simulink model "Working_Dynamics_Sparkle"  (R2018b)
settings: Solver=FixedStepAuto  StartTime=0.0  StopTime=inf  FixedStep=0.0005  RelTol=1e-3
model workspace (MAT data in the model file):
  A_mu = 10
  B_reff = 8.386
  Cz = 7766.25
  DCT_Param.Transmission.Ratios = [3.78 2.18 1.43 1.03 0.935 0.84]
  DCT_Param.Transmission.Shaft_Inertia_Odd = 0.0023
  DCT_Param.Transmission.Shaft_Inertia_Even = 0.0009
  DCT_Param.Transmission.Shaft_Inertia_Output = 0.008
  DCT_Param.Transmission.Gear_Inertia = 0.001
  DCT_Param.Transmission.Gear_Efficiency = 0.94
  DCT_Param.Transmission.Gear_Ang_Vel_Thr = 0.01
  DCT_Param.Transmission.Shaft_Velocity_Odd = 0
  DCT_Param.Transmission.Shaft_Velocity_Even = 0
  DCT_Param.Transmission.Shaft_Velocity_Output = 0
  DCT_Param.Transmission.Gear_Initial_Velocity = 0
  DCT_Param.Transmission.Abstract.Compliance = 100000
  DCT_Param.Transmission.Abstract.Damping = 10000
  DCT_Param.Transmission.Abstract.Ratio_Time_Const = 0.05
  DCT_Param.Transmission.Abstract.Shift_Gear_Delay = 25
  DCT_Param.Clutch.Torque_Radius = 130
  DCT_Param.Clutch.Num_Friction_Surfaces = 4
  DCT_Param.Clutch.Engagement_Piston_Area = 0.001
  DCT_Param.Clutch.Kinetic_Friction_Coeff = 0.3
  DCT_Param.Clutch.Static_Friction_Coeff = 0.31
  DCT_Param.Clutch.Derating_Factor = 1
  DCT_Param.Clutch.Clutch_Velocity_Tolerance = 0.001
  DCT_Param.Clutch.Threshold_Pressure = 1
  DCT_Param.Clutch.Drag_Torque_Coeff = 0
  DCT_Param.Dog_Clutch.Max_Torque = 1000
  DCT_Param.Dog_Clutch.Teeth_Mean_Radius = 50
  DCT_Param.Dog_Clutch.Tooth_Height = 10
  DCT_Param.Dog_Clutch.Ring_Hub_Clearance = 3
  DCT_Param.Dog_Clutch.Ring_Stop_Stiffness = 1000000
  DCT_Param.Dog_Clutch.Ring_Stop_Damping = 1000
  DCT_Param.Dog_Clutch.Shift_Linkage_Damping = 100
  DCT_Param.Dog_Clutch.Max_Engage_Velocity = 1000000
  DCT_Param.Dog_Clutch.Tooth_Engage_Overlap = 3
  DCT_Param.Vehicle.Mass = 1600
  DCT_Param.Vehicle.Wheels_Per_Axle = 2
  DCT_Param.Vehicle.Distance_CG_FrontAxle = 1.7
  DCT_Param.Vehicle.Distance_CG_RearAxle = 2
  DCT_Param.Vehicle.Distance_CG_Ground = 0.5
  DCT_Param.Vehicle.Frontal_Area = 3
  DCT_Param.Vehicle.Aero_Drag_Coeff = 0.4
  DCT_Param.Vehicle.Initial_Velocity = 0
  DCT_Param.Vehicle.Final_Drive_Ratio = 3.7
  DCT_Param.Vehicle.Final_Drive_Efficiency = 0.86
  DCT_Param.Vehicle.Final_Drive_Vel_Thresh = 0.01
  DCT_Param.Vehicle.Side_Shaft_Inertia = 0.01
  DCT_Param.Vehicle.Side_Shaft_Initial_Velocity = 0
  DCT_Param.Vehicle.Tire.Radius = 0.312
  DCT_Param.Vehicle.Tire.Inertia = 0.5
  DCT_Param.Vehicle.Tire.Initial_Velocity = 0
  DCT_Param.Vehicle.Tire.Slip_Vel_Thresh = 0.1
  DCT_Param.Vehicle.Tire.Nominal_Vertical_Load = 4000
  DCT_Param.Vehicle.Tire.C_Coeff = 1.685
  DCT_Param.Vehicle.Tire.D_Coeff = [1.21 -0.037]
  DCT_Param.Vehicle.Tire.E_Coeff = [0.344 0.095 -0.02 0]
  DCT_Param.Vehicle.Tire.BCD_Coeff = [21.51 -0.163 0.245]
  DCT_Param.Vehicle.Tire.H_Coeff = [-0.002 0.002]
  DCT_Param.Vehicle.Tire.V_Coeff = [0 0]
  DCT_Param.ICE.Max_Power = 100000
  DCT_Param.ICE.Speed_At_Max_Power = 5500
  DCT_Param.ICE.Max_Speed = 7000
  DCT_Param.ICE.Stall_Speed = 200
  DCT_Param.ICE.Shaft_Inertia = 0.2
  DCT_Param.ICE.Initial_Velocity = 800
  DCT_Param.ICE.Idle_Ref_Spd = 800
  DCT_Param.ICE.Engine_Time_Constant = 0.2
  DCT_Param.ICE.Initial_Normalized_Throttle = 0
  DCT_Param.ICE.Speed_Threshold = 20
  DCT_Param.ICE.FC.Speed_Vector = [0 368.421052632 736.842105263 1105.26315789 1473.68421053 1842.10526316 2210.52631579 2578.94736842 2947.36842105 3315.78947368 3684.21052632 4052.63157895 4421.05263158 4789.47368421 5157.89473684 5526.31578947 5894.73684211 6263.15789474 6631.57894737 7000]
  DCT_Param.ICE.FC.Torque_Vector = [0 10.5263157895 21.0526315789 31.5789473684 42.1052631579 52.6315789474 63.1578947368 73.6842105263 84.2105263158 94.7368421053 105.263157895 115.789473684 126.315789474 136.842105263 147.368421053 157.894736842 168.421052632 178.947368421 189.473684211 200]
  DCT_Param.ICE.FC.Consumption_Table = [0.262945178015 0.225304787522 0.201465019624 0.191425874321 0.195187351614 0.212749451502 0.244112173984 0.289275519063 0.348239486736 0.421004077004 0.507569289868 0.607935125326 ... (400 elements, 20x20)]
  DCT_Param.Shift_Map_Example.Pedal_Positions = [0.1 0.4 0.5 0.9]
  DCT_Param.Shift_Map_Example.Upshift_Speeds = [11  20  26  34.5  43; 14  26  35  44.5  55; 17  31  42  52.5  65; 21  39  52  66.5  80]
  DCT_Param.Shift_Map_Example.Downshift_Speeds = [8.9  17  23.6  32.4  40.8; 11.5  22.7  32  41.6  52.2; 14  27  38.1  50  62; 18  33  48  62.6  76.2]
  DCT_Param.Shift_Map_ORIG.Pedal_Positions = [0.1 0.4 0.5 0.9]
  DCT_Param.Shift_Map_ORIG.Upshift_Speeds = [11.5  23.5  35.5  45.5  55.5; 14.5  26.5  38.5  48.5  58.5; 17.5  29.5  41.5  51.5  61.5; 20.5  32.5  44.5  54.5  64.5]
  DCT_Param.Shift_Map_ORIG.Downshift_Speeds = [8.5  20.5  32.5  42.5  52.5; 11.5  23.5  35.5  45.5  55.5; 14.5  26.5  38.5  48.5  58.5; 17.5  29.5  41.5  51.5  61.5]
  DCT_Param.Shift_Map_OPT.Pedal_Positions = [0.1 0.4 0.5 0.9]
  DCT_Param.Shift_Map_OPT.Upshift_Speeds = [17.8469  29.8469  35.8159  41.2981  46.3004; 19.2469  33.9778  43.9778  53.9778  63.9778; 24.5469  41.9778  62.1778  78.5778  106.9778; 27.5469  59.3778  99.0445  109.0445  119.0445]
  DCT_Param.Shift_Map_OPT.Downshift_Speeds = [14.8469  26.8469  32.8159  38.2981  43.3004; 16.2469  30.9778  40.9778  50.9778  60.9778; 21.5469  38.9778  59.1778  75.5778  103.9778; 24.5469  56.3778  96.0445  106.0445  116.0445]
  DCT_Param.Shift_Map.Pedal_Positions = [0.1 0.4 0.5 0.9]
  DCT_Param.Shift_Map.Upshift_Speeds = [11.5  23.5  35.5  45.5  55.5; 14.5  26.5  38.5  48.5  58.5; 17.5  29.5  41.5  51.5  61.5; 20.5  32.5  44.5  54.5  64.5]
  DCT_Param.Shift_Map.Downshift_Speeds = [8.5  20.5  32.5  42.5  52.5; 11.5  23.5  35.5  45.5  55.5; 14.5  26.5  38.5  48.5  58.5; 17.5  29.5  41.5  51.5  61.5]
  DCT_Param.Control.Clutch.Min_Lock_Pressure = 2000000
  DCT_Param.Control.Clutch.Max_Lock_Pressure = 5000000
  DCT_Param.Control.Clutch.Max_Unlock_Pressure = 500000
  DCT_Param.Control.Engine_Start_RPM = 800
  DCT_Param.Control.Engine_Stop_RPM = 790
  DCT_Param.Control.Mode_Logic_TS = 0.1
  DCT_Param.Control.ICE.Kp = 0.02
  DCT_Param.Control.ICE.Ki = 0.01
  DCT_Param.Control.Gen.Kp = 10
  DCT_Param.Control.Gen.Ki = 3
  DCT_Param.Control.Mot.Kp = 500
  DCT_Param.Control.Mot.Ki = 300
  DCT_Param.Control.Veh_Spd.Kp = 0.02
  DCT_Param.Control.Veh_Spd.Ki = 0.04
  DCT_Param.Driver.Kp = 400
  DCT_Param.Driver.Ki = 0.001
  DCT_Param.Driver.Pedal_Filter_Const = 0.01
  DCT_Param.Dog_Clutches.Pulse_Delay = 50
  DCT_Param.Dog_Clutches.Pulse_Length = 20
  DCT_Param.Animation.Teeth_Ratios = [0.338461538462 0.555555555556 0.916666666667 0.96 1.17948717949 1.92307692308]
  DCT_Param.Animation.Teeth_Ratios_Reverse = [0.458333333333 0.75]
  DCT_Param.Shift_Map_OPT506.Pedal_Positions = [0.1 0.4 0.5 0.9]
  DCT_Param.Shift_Map_OPT506.Upshift_Speeds = [18  30.2  48.3  67.3322  77.3429; 20.1  36.85  66.6178  76.7537  86.7537; 21.1  40.25  71.0189  81.0189  91.7873; 24.1  63.75  80.7523  105.9489  115.9489]
  DCT_Param.Shift_Map_OPT506.Downshift_Speeds = [15  27.2  45.3  64.3322  74.3429; 17.1  33.85  63.6178  73.7537  83.7537; 18.1  37.25  68.0189  78.0189  88.7873; 21.1  60.75  77.7523  102.9489  112.9489]
  DCT_Param.Shift_Map_OPTAbsRea176.Pedal_Positions = [0.1 0.4 0.5 0.9]
  DCT_Param.Shift_Map_OPTAbsRea176.Upshift_Speeds = [17.8469  29.8469  35.7875  44.0901  49.4243; 18.9219  34.1312  45.8256  59.7585  69.7585; 32.1719  43.4585  53.51  103.2151  114.6401; 35.1719  59.2585  99.5217  109.5217  119.5217]
  DCT_Param.Shift_Map_OPTAbsRea176.Downshift_Speeds = [14.8469  26.8469  32.7875  41.0901  46.4243; 15.9219  31.1312  42.8256  56.7585  66.7585; 29.1719  40.4585  50.51  100.2151  111.6401; 32.1719  56.2585  96.5217  106.5217  116.5217]
  D_reff = 0.25826
  Downshift_Speeds = [9.5625  23.0625  36.5625  47.8125  59.0625  68.90625  78.75; 12.9375  26.4375  39.9375  51.1875  62.4375  72.84375  83.25; 16.3125  29.8125  43.3125  54.5625  65.8125  76.78125  87.75; 19.6875  33.1875  46.6875  57.9375  69.1875  80.71875  92.25]
  Pedal_Positions = [0.1 0.4 0.5 0.9]
  SUS.Stiffness = 24000
  SUS.Damping.Constant = 1262
  SUS.Damping.Rebound = [4040 4950 2883 2043]
  SUS.Damping.Compression = [3600 3420 1863 1472]
  SUS.PistonSpeed = [0.05 0.1 0.3 0.6]
  SUS.UnsprungMass.Fr = 21.0693333333
  SUS.UnsprungMass.Rr = 21.0693333333
  Upshift_Speeds = [12.9375  26.4375  39.9375  51.1875  62.4375  72.84375  83.25; 16.3125  29.8125  43.3125  54.5625  65.8125  76.78125  87.75; 19.6875  33.1875  46.6875  57.9375  69.1875  80.71875  92.25; 33  52.5  77.25  100.5  138.75  161.875  185]
  VEH.Mass = 1181
  VEH.StaticNormalFrontLoad.FR = 264.666666667
  VEH.StaticNormalFrontLoad.FL = 264.666666667
  VEH.StaticNormalRearLoad.RR = 322
  VEH.StaticNormalRearLoad.RL = 322
  VEH.WheelBase = 3.075
  VEH.FrontAxlePositionfromCG = 1.515
  VEH.RearAxlePositionfromCG = 1.504
  VEH.HeightCG = 0.134
  VEH.FrontalArea = 2.11
  VEH.DragCoefficient = 0.33
  VEH.NumberOfWheelsPerAxle = 2
  VEH.Thread.FR = 1.705
  VEH.Thread.RR = 1.705
  VEH.PitchMomentInertia = 1922.66666667
  VEH.RollMomentInertia = 432.333333333
  VEH.YawMomentInertia = 2066
  VEH.SteeringRatio = 18
  VEH.TrackWidth = 1.922
  VEH.SprungMass = 1096.72266667
  VEH.InitialLongPosition = 0
  VEH.InitialLatPosition = 3.125
  VEH.InitialVertPosition = 0.0111
  VEH.InitialRollAngle = 0
  VEH.InitialPitchAngle = -0.000732
  VEH.InitialYawAngle = 0
  VEH.InitialLongVel = 0
  VEH.InitialLatVel = 0
  VEH.InitialVertVel = 0
  VEH.InitialRollRate = 0
  VEH.InitialPitchRate = 0
  VEH.InitialYawRate = 0
  V_o = 16.7
  V_xlow = 1
  WH.Tire.Radius.Front = 0.384
  WH.Tire.Radius.Rear = 0.401
  WH.Tire.Sidewall = 0.245
  WH.Tire.RollingResistCoeff = 0.0103
  WH.Tire.Magic.B = 10
  WH.Tire.Magic.C = 1.9
  WH.Tire.Magic.D = 1
  WH.Tire.Magic.E = 0.97
  WH.Tire.Magic.Bx = 12
  WH.Tire.Magic.Cx = 1.9
  WH.Tire.Magic.Dx = 0.72
  WH.Tire.Magic.Ex = 0.95
  WH.Tire.Magic.By = 12
  WH.Tire.Magic.Cy = 1.3
  WH.Tire.Magic.Dy = 0.75
  WH.Tire.Magic.Ey = 0.2
  WH.Tire.Front.Ky = 40000
  WH.Tire.Rear.Ky = 40000
  WH.Tire.Kz = 320000
  WH.Tire.Damping = 100
  WH.Inertia = 1.00333333333
  WH.Mass = 11.4333333333
  WH.DampingCoefficient = 0.01
  WH.VelocityTol = 0.1
  a = 1.4
  alpha_max = 1.5
  alpha_min = -1.5
  b = 1.8
  c_zo = 209651
  epsilon = 0.1
  h = 0.134
  path.ISO3888p2.x = [0 2 12 25.5 36.5 49 61]
  path.ISO3888p2.y = [0 0 0 3.725 3.725 0 0]
  path.ISO3888p2.ylb = [1.225 1.225 1.225 4.725 4.725 1.5 1.5]
  path.ISO3888p2.yrb = [-1.225 -1.225 -1.225 2.225 2.225 -1.5 -1.5]
  path.CUSC.x = [10.668 21.336 36.576 54.864 73.152]
  path.CUSC.y = [0 0 5.1816 0 0]
  path.CUSC.ylb = [1.2192 1.2192 7.0104 1.8288 1.8288]
  path.CUSC.yrb = [-1.2192 -1.2192 3.3528 -1.8288 -1.8288]
  pio = 220000
  q_Fcx = 0
  q_Fz2 = 15.4
  q_Fzy = 0
  q_reo = 0.9974
  q_sx1 = -0.007764
  q_sx10 = 0.2824
  q_sx11 = 5.349
  q_sx12 = 0
  q_sx13 = 0
  q_sx14 = 0
  q_sx2 = 1.1915
  q_sx3 = 0.013948
  q_sx4 = 4.912
  q_sx5 = 1.02
  q_sx6 = 22.83
  q_sx7 = 0.7104
  q_sx8 = -0.023393
  q_sx9 = 0.6581
  q_sy1 = 0.00702
  q_sy2 = 0
  q_sy3 = 0.001515
  q_sy4 = 8.514e-05
  q_sy5 = 0
  q_sy6 = 0
  q_sy7 = 0.9008
  q_sy8 = -0.4089
  q_v1 = 0.0007742
  q_v2 = 0.04667
  r_Bx1 = 12.531
  r_Bx2 = 9.532
  r_Bx3 = 0
  r_By1 = 10.615
  r_By2 = 7.705
  r_By3 = 3.433e-06
  r_By4 = 0
  r_Cx1 = 1.019
  r_Cy1 = 1.0585
  r_Ex1 = -0.4487
  r_Ex2 = -0.4726
  r_Ey1 = 0.3132
  r_Ey2 = 7.63e-06
  r_Hx1 = 0.0002374
  r_Hy1 = 0.011646
  r_Hy2 = 7.63e-06
  r_Vy1 = 0.05654
  r_Vy2 = 7.63e-06
  r_Vy3 = 0
  r_Vy4 = 99.9
  r_Vy5 = 2
  r_Vy6 = 15.814
  r_o = 0.3135
  vehWidth = 2
  w = 1
libraries: robotlib x13, autolibutils x8, autolibshared x6, simulink x6, sim3dlib x3, autolibsharedcoupling x3, vehdynlibtirecommon x2, vehdynlibsteering x1, autolibshareddiff x1, autolibsharedtransfixedgear x1, sharedtransform x1, autolibsharedmappedengines x1
(part 1 of 6)
settings Model: Creator=ivory  LastModifiedBy=ivory
settings OptimizationCC: EnhancedBackFolding=on  PassReuseOutputArgsAs=Individual arguments  MaxStackSize=64  OptimizeBlockOrder=speed  DifferentSizesBufferReuse=on
settings DebuggingCC: SignalInfNanChecking=warning  ParameterTunabilityLossMsg=error  UnderSpecifiedDimensionMsg=error
settings HardwareCC: ProdBitPerPointer=32  ProdBitPerSizeT=32  ProdBitPerPtrDiffT=32  ProdLargestAtomicFloat=None  ProdIntDivRoundTo=Undefined  ProdEndianess=Unspecified  ProdWordSize=32  ProdHWDeviceType=Generic->Unspecified (assume 32-bit Generic)
settings ModelReferenceCC: ModelReferenceMinAlgLoopOccurrences=on
settings SFSimCC: MATLABDynamicMemAlloc=off
settings RTWCC: SystemTargetFile=ert.tlc  HardwareBoard=Robot Operating System (ROS)  TLCOptions="-aInlineSetEventsForThisBaseRateFcn=TLC_FALSE -aSuppressMultiTaskScheduler=TLC_FALSE  -aRateBasedStepFcn=0"  TemplateMakefile=ert_default_tmf  GenerateReport=on  Toolchain=Catkin  IncludeHyperlinkInReport=on  LaunchReport=on  TargetLang=C++  GenerateTraceInfo=on  GenerateTraceReport=on  GenerateTraceReportSl=on  GenerateTraceReportSf=on  GenerateTraceReportEml=on  GenerateCodeMetricsReport=on
settings CodeAppCC: ForceParamTrailComments=on  IgnoreCustomStorageClasses=off  OperatorAnnotations=on  SimulinkDataObjDesc=on  SFDataObjDesc=on  InsertBlockDesc=on
settings ERTTargetCC: SupportContinuousTime=on  SupportVariableSizeSignals=on

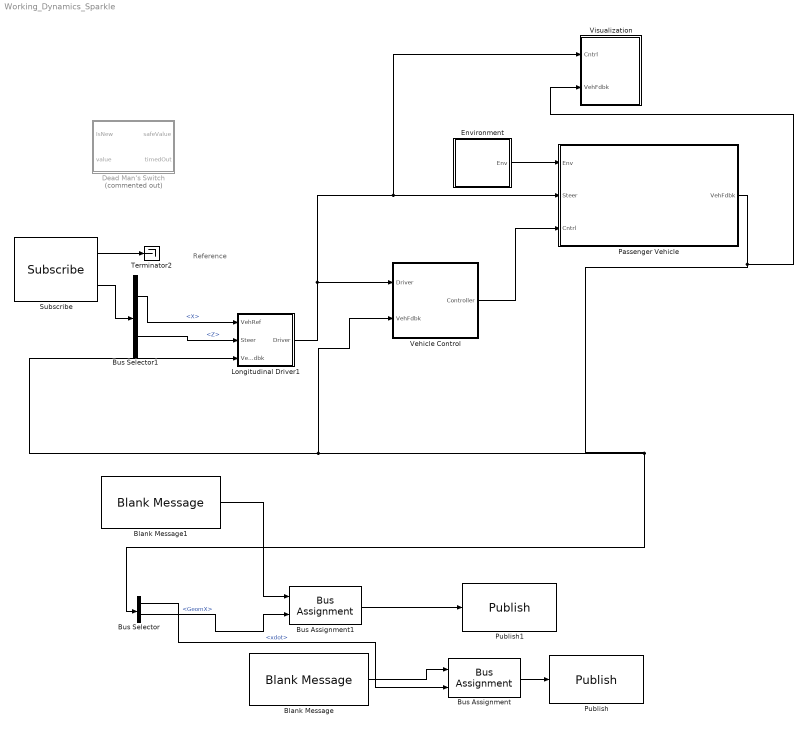
== system Working_Dynamics_Sparkle ==
  note: Reference
  Blank Message : robotlib/Blank Message  messageClass=Message  entityType=geometry_msgs/Twist  messageType=geometry_msgs/Twist  SampleTime=inf
      settings: SourceProductBaseCode=RO
  Blank Message1 : robotlib/Blank Message  messageClass=Message  entityType=std_msgs/Float64  messageType=std_msgs/Float64  SampleTime=inf
      settings: SourceProductBaseCode=RO
  Bus Assignment : BusAssignment  AssignedSignals=Linear.X
  Bus Assignment1 : BusAssignment  AssignedSignals=Data
  Bus Selector : BusSelector  OutputSignals=Body.xdot,Body.GeomX
  Bus Selector1 : BusSelector  OutputSignals=Linear.X,Angular.Z
  Dead Man's Switch : Subsystem  Commented=on  TreatAsAtomicUnit=on  mask{stepSize=0.001, timeout=0.2}
      mask prompts: stepSize "Simulation step size"; timeout "Timeout (in seconds)"
      mask help: Interprets whether a new message has been recently received, and if so permits the data in 'value' to be passed through. Otherwise, 0 is outputted from 'safeValue'
      mask Help: Interprets whether a new message has been recently received, and if so permits the data in 'value' to be passed through. Otherwise, 0 is outputted from 'safeValue'
  Environment : Subsystem
      mask Display: disp('Environment')
  Longitudinal Driver1 : Subsystem  VariantControl=0
      mask Display: image('longitudinal_driver_pedals.png');
  Passenger Vehicle : Subsystem
      mask Display: image('/home/ivory/VersionControl/rahulbhadani.github.io/images/carlogo.png');
  Publish : robotlib/Publish  topicSource=Specify your own  topic=/catvehicle/vel  messageType=geometry_msgs/Twist  messageQueueLength=1
      settings: SourceProductBaseCode=RO
  Publish1 : robotlib/Publish  topicSource=Specify your own  topic=/catvehicle/X  messageType=std_msgs/Float64  messageQueueLength=1
      settings: SourceProductBaseCode=RO
  Subscribe : robotlib/Subscribe  topicSource=Specify your own  topic=/catvehicle/cmd_vel  messageType=geometry_msgs/Twist  sampleTime=-1  messageQueueLength=1
      settings: SourceProductBaseCode=RO
  Terminator2 : Terminator
  Vehicle Control : Subsystem
      mask Display: image('/home/ivory/Pictures/actuator.jpg');
  Visualization : Subsystem
      mask Display: disp('Visualization')
  wires:
  Bus Selector1/1 -> Longitudinal Driver1/1(VehRef)  "<X>"
  Subscribe/1 -> Terminator2/1
  Subscribe/2 -> Bus Selector1/1
  Bus Assignment/1 -> Publish/1
  Bus Selector1/2 -> Longitudinal Driver1/2(Steer)  "<Z>"
  Blank Message/1 -> Bus Assignment/1
  Environment/1(Env) -> Passenger Vehicle/1(Env)
  Vehicle Control/1(Controller) -> Passenger Vehicle/3(Cntrl)
  Bus Assignment1/1 -> Publish1/1
  Bus Selector/2 -> Bus Assignment1/2  "<GeomX>"
  Blank Message1/1 -> Bus Assignment1/1
  Bus Selector/1 -> Bus Assignment/2  "<xdot>"
  Longitudinal Driver1/1(Driver) -> Visualization/1(Cntrl), Passenger Vehicle/2(Steer), Vehicle Control/1(Driver)
  Passenger Vehicle/1(VehFdbk) -> Visualization/2(VehFdbk), Bus Selector/1, Longitudinal Driver1/3(VehFdbk), Vehicle Control/2(VehFdbk)

== system Working_Dynamics_Sparkle/Dead Man's Switch ==
  note: The timeout value, and step size, are critical to set correctly here.
  IsNew : Inport
  value : Inport  Port=2
  Simulate step size : Constant  Value=stepSize
  Timeout in seconds : Constant  Value=timeout
  timeout set to 0 output : MATLAB Function  TreatAsAtomicUnit=on
  safeValue : Outport  InitialOutput=[0]
  timedOut : Outport  Port=2  InitialOutput=[0]
  wires:
  IsNew/1 -> timeout set to 0 output/1(isNew)
  timeout set to 0 output/1(safeValue) -> safeValue/1
  value/1 -> timeout set to 0 output/2(value)
  Timeout in seconds/1 -> timeout set to 0 output/3(timeout)
  timeout set to 0 output/2(timedOut) -> timedOut/1
  Simulate step size/1 -> timeout set to 0 output/4(stepSize)

== system Working_Dynamics_Sparkle/Environment ==
  Bus Creator1 : BusCreator  Inputs=2
  Constant3 : Constant  Value=0
  Constant4 : Constant  Value=0
  Constant5 : Constant  Value=0
  Friction : Constant  Value=ones(4,1).*1.0
  Ground Feedback : Subsystem  VariantControlMode=Label  Variant=on  LabelModeActiveChoice=0
  Vector Concatenate : Concatenate  NumInputs=3
  Env : Outport
  wires:
  Constant5/1 -> Vector Concatenate/3  "Z"
  Vector Concatenate/1 -> Bus Creator1/1  "Wind"
  Constant3/1 -> Vector Concatenate/1  "X"
  Constant4/1 -> Vector Concatenate/2  "Y"
  Ground Feedback/1(Ground) -> Bus Creator1/2  "Gnd"
  Bus Creator1/1 -> Env/1
  Friction/1 -> Ground Feedback/1(Friction)

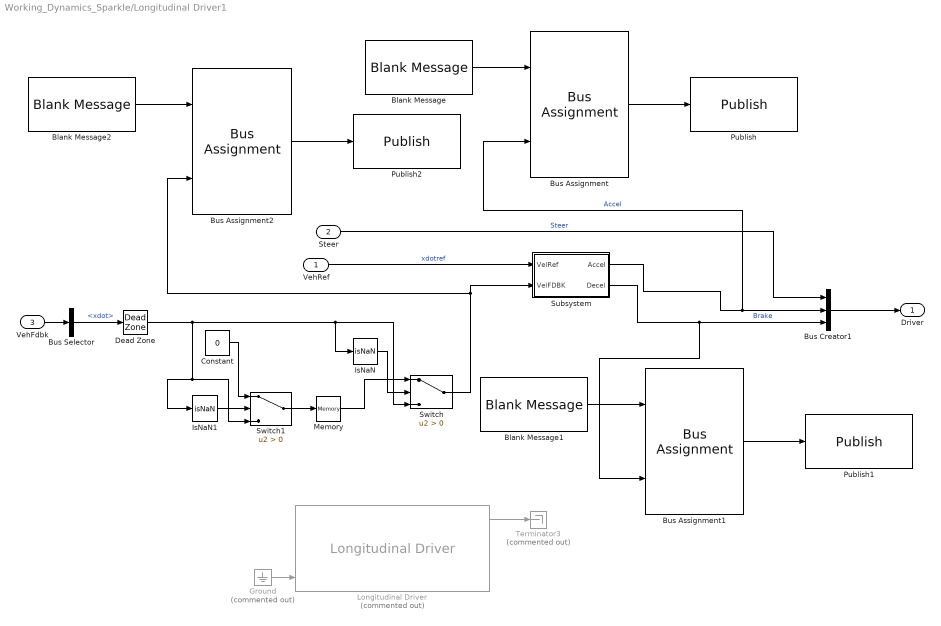
== system Working_Dynamics_Sparkle/Longitudinal Driver1 ==
  VehRef : Inport  Unit=m/s
  Steer : Inport  Port=2  Unit=rad
  VehFdbk : Inport  Port=3
  Blank Message : robotlib/Blank Message  messageClass=Message  entityType=std_msgs/Float64  messageType=std_msgs/Float64  SampleTime=inf
      settings: SourceProductBaseCode=RO
  Blank Message1 : robotlib/Blank Message  messageClass=Message  entityType=std_msgs/Float64  messageType=std_msgs/Float64  SampleTime=inf
      settings: SourceProductBaseCode=RO
  Blank Message2 : robotlib/Blank Message  messageClass=Message  entityType=std_msgs/Float64  messageType=std_msgs/Float64  SampleTime=inf
      settings: SourceProductBaseCode=RO
  Bus Assignment : BusAssignment  AssignedSignals=Data
  Bus Assignment1 : BusAssignment  AssignedSignals=Data
  Bus Assignment2 : BusAssignment  AssignedSignals=Data
  Bus Creator1 : BusCreator  Inputs=3
  Bus Selector : BusSelector  OutputSignals=Body.xdot
  Constant : Constant  Value=0
  Dead Zone : DeadZone  LowerValue=-0.0001  UpperValue=0.0001  SaturateOnIntegerOverflow=on
  Ground : Ground  Commented=on
  IsNaN : RelationalOperator  Operator=isNaN  OutDataTypeStr=boolean  RndMeth=Simplest
  IsNaN1 : RelationalOperator  Operator=isNaN  OutDataTypeStr=boolean  RndMeth=Simplest
  Longitudinal Driver : autolibshared/Longitudinal Driver  Commented=on  cntrlType=Predictive  shftType=None  velUnits=m/s  gearOut=off  Kp=8  Ki=5  Kff=0.5  Kg=0  VehVelVec=[0 100]  KffVec=[.1 .1]  KpVec=[10 10]  KiVec=[5 5]  KgVec=[0 0]  m=1700  Kpt=3000  tau=.10  L=5  aR=200  bR=2.5  cR=.25  g=9.81  vnom=1.0  Kaw=1  tauerr=.075  tauPt=2  GearInit=0  tShift=.1  pdlVec=[0.1 0.4 0.5 0.9]  upShftTbl=[-1 12.9375 26.4375 39.9375 51.18749999999999 62.4375 72.84375 83.25;-1 16.3125 29.8125 43.3125 54.5624 65.8125 76.78125 87.75;-1 19.6875 33.1875 46.68749999999999 57.9375 69.1875 80.71875 92.25;-1 33 52.5 77.25 100.5 138.75 161.875 185]  dwnShftTbl=[1 9.5625 23.0625 36.5625 47.8125 59.0625 68.90625 78.75;1 12.9375 26.4375 39.9375 51.18749999999999 62.4375 72.84375 83.25;1 16.3125 29.8125 43.3125 54.562499 65.8125 76.78125 87.75;1 19.6875 33.1875 46.68749999999999 57.9375 69.1875 80.71875 92.25]  tClutch=.5  tRev=.5  tPark=120  aMode=2  UpGearVec="[0  1  2  3  4  5  6  7]"  DownGearVec="[1  2  3  4  5  6  7  8]"
      settings: SourceProductName=Powertrain Blockset  SourceProductBaseCode=PW
  Memory : Memory  InheritSampleTime=on  LinearizeAsDelay=on
  Publish : robotlib/Publish  topicSource=Specify your own  topic=/catvehicle/accel_in  messageType=std_msgs/Float64  messageQueueLength=1
      settings: SourceProductBaseCode=RO
  Publish1 : robotlib/Publish  topicSource=Specify your own  topic=/catvehicle/brake_in  messageType=std_msgs/Float64  messageQueueLength=1
      settings: SourceProductBaseCode=RO
  Publish2 : robotlib/Publish  topicSource=Specify your own  topic=/catvehicle/v_feed  messageType=std_msgs/Float64  messageQueueLength=1
      settings: SourceProductBaseCode=RO
  Subsystem : Subsystem
  Switch : Switch  Criteria=u2 > Threshold
  Switch1 : Switch  Criteria=u2 > Threshold
  Terminator3 : Terminator  Commented=on
  Driver : Outport
  wires:
  Subsystem/2(Decel) -> Bus Assignment1/2, Bus Creator1/3  "Brake"
  Ground/1 -> Longitudinal Driver/3
  Subsystem/1(Accel) -> Bus Assignment/2, Bus Creator1/2  "Accel"
  VehFdbk/1 -> Bus Selector/1
  Bus Creator1/1 -> Driver/1
  VehRef/1 -> Subsystem/1(VelRef)  "xdotref"
  Longitudinal Driver/1 -> Terminator3/1
  Dead Zone/1 -> Switch/3, IsNaN/1, IsNaN1/1, Switch1/3
  Steer/1 -> Bus Creator1/1  "Steer"
  Blank Message/1 -> Bus Assignment/1
  Bus Assignment/1 -> Publish/1
  Bus Assignment1/1 -> Publish1/1
  Blank Message1/1 -> Bus Assignment1/1
  Bus Assignment2/1 -> Publish2/1
  Blank Message2/1 -> Bus Assignment2/1
  IsNaN/1 -> Switch/2
  Memory/1 -> Switch/1
  Switch/1 -> Subsystem/2(VelFDBK), Bus Assignment2/2
  IsNaN1/1 -> Switch1/2
  Constant/1 -> Switch1/1
  Switch1/1 -> Memory/1
  Bus Selector/1 -> Dead Zone/1  "<xdot>"

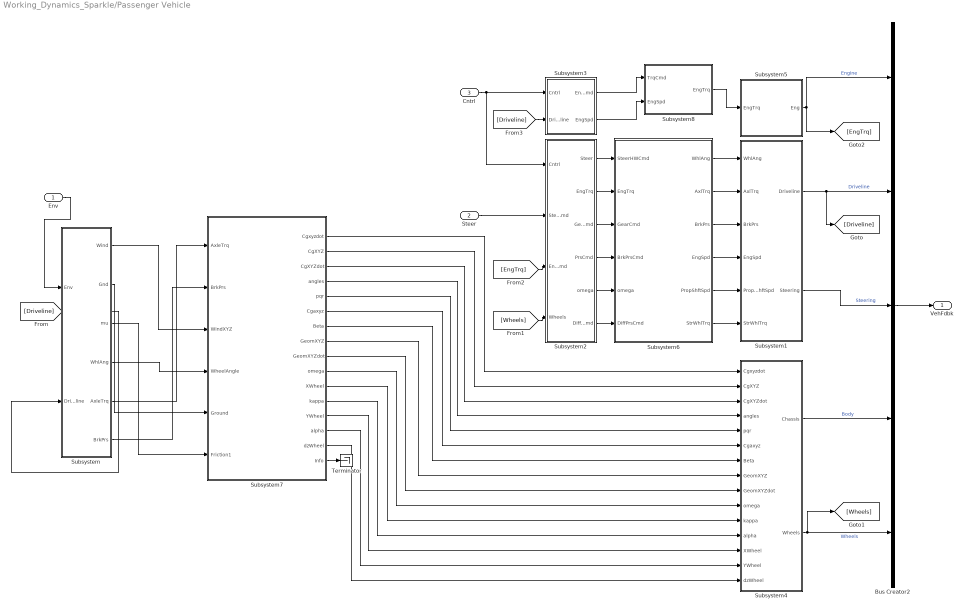
== system Working_Dynamics_Sparkle/Passenger Vehicle ==
  Env : Inport
  Steer : Inport  Port=2
  Cntrl : Inport  Port=3
  Bus Creator2 : BusCreator  Inputs=5
  Subsystem : Subsystem
  Subsystem1 : Subsystem
  Subsystem2 : Subsystem
  Subsystem3 : Subsystem
  Subsystem4 : Subsystem
  Subsystem5 : Subsystem
  Subsystem6 : Subsystem
  Subsystem7 : Subsystem
  Subsystem8 : Subsystem
  Terminator : Terminator
  VehFdbk : Outport
  wires:
  Bus Creator2/1 -> VehFdbk/1
  Env/1 -> Subsystem/1(Env)
  Subsystem1/1(Driveline) -> [Driveline], Bus Creator2/2  "Driveline"
  Subsystem6/1(WhlAng) -> Subsystem1/1(WhlAng)
  Subsystem6/2(AxlTrq) -> Subsystem1/2(AxlTrq)
  Subsystem6/3(BrkPrs) -> Subsystem1/3(BrkPrs)
  Subsystem6/4(EngSpd) -> Subsystem1/4(EngSpd)
  Subsystem6/5(PropShftSpd) -> Subsystem1/5(PropShftSpd)
  Steer/1 -> Subsystem2/2(SteerCmd)
  Cntrl/1 -> Subsystem2/1(Cntrl), Subsystem3/1(Cntrl)
  Subsystem8/1(EngTrq) -> Subsystem5/1("EngTrq ")
  Subsystem3/1(EngTrqCmd) -> Subsystem8/1(TrqCmd)
  Subsystem3/2(EngSpd) -> Subsystem8/2(EngSpd)
  Subsystem4/1(Chassis) -> Bus Creator2/4  "Body"
  Subsystem4/2(Wheels) -> [Wheels], Bus Creator2/5  "Wheels"
  Subsystem5/1(Eng) -> [EngTrq], Bus Creator2/1  "Engine"
  [Driveline] -> Subsystem/2(Driveline)
  [Wheels] -> Subsystem2/4(Wheels)
  [EngTrq] -> Subsystem2/3(EngTrqCmd)
  [Driveline] -> Subsystem3/2(Driveline)
  Subsystem/6(BrkPrs) -> Subsystem7/2(BrkPrs)
  Subsystem/3(mu) -> Subsystem7/6(Friction1)
  Subsystem/4(WhlAng) -> Subsystem7/4(WheelAngle)
  Subsystem/1(Wind) -> Subsystem7/3(WindXYZ)
  Subsystem/2(Gnd) -> Subsystem7/5(Ground)
  Subsystem/5(AxleTrq) -> Subsystem7/1(AxleTrq)
  Subsystem2/6(DiffPrsCmd) -> Subsystem6/6(DiffPrsCmd)
  Subsystem2/2(EngTrq) -> Subsystem6/2(EngTrq)
  Subsystem2/4(PrsCmd) -> Subsystem6/4(BrkPrsCmd)
  Subsystem2/1(Steer) -> Subsystem6/1(SteerHWCmd)
  Subsystem2/3(GearCmd) -> Subsystem6/3(GearCmd)
  Subsystem2/5(omega) -> Subsystem6/5(omega)
  Subsystem6/6(StrWhlTrq) -> Subsystem1/6(StrWhlTrq)
  Subsystem1/2(Steering) -> Bus Creator2/3  "Steering"
  Subsystem7/12(kappa) -> Subsystem4/12(alpha)
  Subsystem7/11(XWheel) -> Subsystem4/11(kappa)
  Subsystem7/13(" YWheel") -> Subsystem4/13(XWheel)
  Subsystem7/2(CgXYZ) -> Subsystem4/2(CgXYZ)
  Subsystem7/15(dzWheel) -> Subsystem4/15(dzWheel)
  Subsystem7/10(omega) -> Subsystem4/10(omega)
  Subsystem7/1(Cgxyzdot) -> Subsystem4/1(Cgxyzdot)
  Subsystem7/8(GeomXYZ) -> Subsystem4/8(GeomXYZ)
  Subsystem7/5(pqr) -> Subsystem4/5(pqr)
  Subsystem7/7(Beta) -> Subsystem4/7(Beta)
  Subsystem7/4(angles) -> Subsystem4/4(angles)
  Subsystem7/3(CgXYZdot) -> Subsystem4/3(CgXYZdot)
  Subsystem7/6(Cgaxyz) -> Subsystem4/6(Cgaxyz)
  Subsystem7/9(GeomXYZdot) -> Subsystem4/9(GeomXYZdot)
  Subsystem7/14(alpha) -> Subsystem4/14(YWheel)
  Subsystem7/16(" Info") -> Terminator/1

== system Working_Dynamics_Sparkle/Vehicle Control ==
  Driver : Inport
  VehFdbk : Inport  Port=2
  Active Differential Control : Subsystem  VariantControlMode=Label  Variant=on  LabelModeActiveChoice=0
  Brake Controller : Subsystem
  Bus Creator{,1..2,4} (4 alike) : BusCreator  Inputs=1
  Bus Creator3 : BusCreator  Inputs=4
  Bus Selector : BusSelector  OutputSignals=Body.xdot,Wheels.kappa,Body.r
  Bus Selector1 : BusSelector  OutputSignals=Driveline.EngSpd,Driveline.PropShftSpd
  Bus Selector2 : BusSelector  OutputSignals=Accel,Brake
  Bus Selector3 : BusSelector  OutputSignals=Steer
  ECU : Subsystem
  Max : MinMax  Function=max  Inputs=2
  Transmission Controller : Subsystem
  Controller : Outport
  wires:
  Transmission Controller/1(Gear) -> Bus Creator1/1  "GearCmd"
  Bus Selector/2 -> Brake Controller/3(kappa)  "<kappa>"
  ECU/1(Trq Cmd) -> Max/1
  Brake Controller/1(PCmd) -> Bus Creator2/1  "PrsCmd"
  VehFdbk/1 -> Bus Selector/1, Bus Selector1/1
  Bus Selector/1 -> Brake Controller/2(xdot)  "<xdot>"
  Bus Selector1/1 -> Transmission Controller/2(EngSpd)  "<EngSpd>"
  Bus Selector1/2 -> Transmission Controller/3(PropShaftSpd)  "<PropShftSpd>"
  Driver/1 -> Bus Selector3/1, Bus Selector2/1
  Bus Selector2/1 -> Transmission Controller/1(Acc), ECU/1(<Accel>)  "<Accel>"
  Bus Selector2/2 -> Brake Controller/1(BrkCmd)  "<Brake>"
  Bus Creator/1 -> Bus Creator3/1  "ECU"
  Bus Creator1/1 -> Bus Creator3/2  "Transmission"
  Bus Creator2/1 -> Bus Creator3/3  "Brake"
  Bus Creator3/1 -> Controller/1  "Controller"
  Bus Creator4/1 -> Bus Creator3/4  "Diff"
  Active Differential Control/1(DiffPrsCmd) -> Bus Creator4/1  "PrsCmd"
  Bus Selector3/1 -> Active Differential Control/2(Steer)  "<Steer>"
  Active Differential Control/2(TrqCmd) -> [DiffTrqCmd]
  Max/1 -> Bus Creator/1  "EngTrqCmd"
  [DiffTrqCmd] -> Max/2
  Bus Selector/3 -> Active Differential Control/1(YawRate)  "<r>"

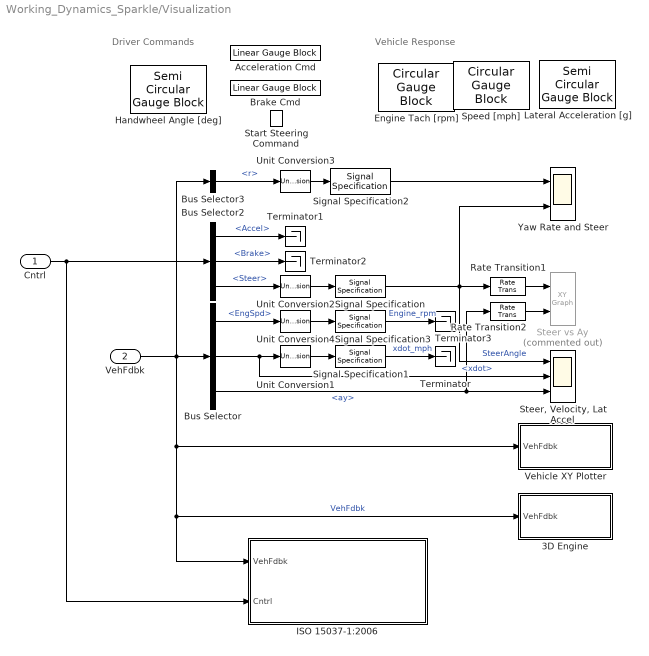
== system Working_Dynamics_Sparkle/Visualization ==
  note: Vehicle Response
  note: Driver Commands
  Cntrl : Inport
  VehFdbk : Inport  Port=2
  3D Engine : Subsystem  VariantControlMode=Label  Variant=on  LabelModeActiveChoice=0  mask(3D Engine){engine3D=Disabled, SceneDesc=Open surface, dt3D=.03}
      mask prompts: engine3D "3D Engine"; SceneDesc "Scene Description:"; dt3D "Engine frame rate, dt3D [s]:"
      mask help: This subsystem contains the interface blocks which permit the display of the vehicle in 3D virtual environment. Enable it to view the simulation progress, disable it to inhibit the display.
      mask init:
      | switch get_param(gcb,'engine3D')
      |     case 'Disabled'
      |         set_param(gcb,'OverrideUsingVariant','0')
      |         try
      |             set_param([bdroot '/Environment/Ground Feedback'],'OverrideUsingVariant','0')
      |         catch
      |             disp('No ground feedback sensor found')
      |         end
      |     case 'Enabled'
      |         set_param(gcb,'OverrideUsingVariant','1')
      |         try
      |             set_param([bdroot '/Environment/Ground Feedback'],'OverrideUsingVariant','1')
      |         catch
      |             disp('No ground feedback sensor found')
      |         end
      |     otherwise
      |         set_param(gcb,'OverrideUsingVariant','0')
      | end
      settings: AttributesFormatString=%<engine3D>
      mask Help: eval('vdynblkshelp(''vdynblksscenecameraray'')');
      mask TypeOptions engine3D: Enabled | Disabled
      mask Callback engine3D:
      | switch get_param(gcb,'engine3D')
      |     case 'Disabled'
      |         set_param(gcb,'OverrideUsingVariant','0')
      |     case 'Enabled'
      |        set_param(gcb,'OverrideUsingVariant','1')
      |     otherwise
      |        set_param(gcb,'OverrideUsingVariant','0')
      | end
      mask TypeOptions SceneDesc:
      | 3D Engine/Simulation 3D Engine
      | 1/SceneDesc
      mask Display: disp('3D Engine')
  Acceleration Cmd : LinearGaugeBlock  WebBlockId=2002  LabelPosition=Hide  ScaleMax=1
  Brake Cmd : LinearGaugeBlock  WebBlockId=2003  LabelPosition=Hide  ScaleMax=1
  Bus Selector : BusSelector  OutputSignals=Driveline.EngSpd,Body.xdot,Body.ay
  Bus Selector2 : BusSelector  OutputSignals=Accel,Brake,Steer
  Bus Selector3 : BusSelector  OutputSignals=Body.r
  Engine Tach [rpm] : CircularGaugeBlock  WebBlockId=2007  LabelPosition=Hide  ScaleMax=8000  TickInterval=1000
  Handwheel Angle [deg] : SemiCircularGaugeBlock  WebBlockId=2008  LabelPosition=Hide  ScaleMin=-300  ScaleMax=300  TickInterval=60
  ISO 15037-1:2006 : Subsystem  StopFcn=|  VariantControlMode=Label  Variant=on  LabelModeActiveChoice=0  mask(ISO 15037-1:2006){Measurement=Disabled}
      | switch get_param(gcb,'Measurement')
      |     case 'Enabled'
      |        p=slproject.getCurrentProject;
      |        projectRoot=p.RootFolder;
      |        SySFolder=fullfile(projectRoot, 'System');
      |        Simulink.sdi.loadView([SySFolder filesep 'ISO15037_1_2006E.mldatx']);
      |        Simulink.sdi.view;
      | end
      mask prompts: Measurement "ISO Measurements"
      mask help: Enables display of ISO 15037-1:2006 standard measurement signals in the Simulation Data Inspector.
      mask init:
      | switch get_param(gcb,'Measurement')
      |     case 'Disabled'
      |         set_param(gcb,'OverrideUsingVariant','0')
      |     case 'Enabled'
      |        set_param(gcb,'OverrideUsingVariant','1')
      |     otherwise
      |        set_param(gcb,'OverrideUsingVariant','0')
      | end
      settings: AttributesFormatString=%<Measurement>
      mask Help: eval('vdynblkshelp(''iso15037'')');
      mask TypeOptions Measurement: Enabled | Disabled
      mask Callback Measurement:
      | switch get_param(gcb,'Measurement')
      |     case 'Disabled'
      |         set_param(gcb,'OverrideUsingVariant','0')
      |     case 'Enabled'
      |        set_param(gcb,'OverrideUsingVariant','1')
      |     otherwise
      |        set_param(gcb,'OverrideUsingVariant','0')
      | end
      mask Display: disp('ISO 15037-1:2006')
  Lateral Acceleration [g] : SemiCircularGaugeBlock  WebBlockId=2058  LabelPosition=Hide  ScaleMin=-1  ScaleMax=1  TickInterval=0.5
  Rate Transition1 : RateTransition  Deterministic=off  OutPortSampleTime=.1
  Rate Transition2 : RateTransition  Deterministic=off  OutPortSampleTime=.1
  Signal Specification : SignalSpecification  Unit=deg
  Signal Specification1 : SignalSpecification  Unit=mph
  Signal Specification2 : SignalSpecification  Unit=deg/s
  Signal Specification3 : SignalSpecification  Unit=rpm
  Speed [mph] : CircularGaugeBlock  WebBlockId=2065  LabelPosition=Hide  TickInterval=10
  Start Steering Command : LampBlock  WebBlockId=2066  LabelPosition=Hide
  Steer vs Ay : simulink/Sinks/XY Graph  Commented=on  xmin=-300  xmax=300  ymin=-1.5  ymax=1.5  st=.1
  "Steer, Velocity, Lat Accel" : Scope  NumInputPorts=3
  Terminator{,1..3} (4 alike) : Terminator
  Unit Conversion{1..4} (4 alike) : UnitConversion
  Vehicle XY Plotter : Subsystem  mask(Vehicle XY Plotter){a=VEH.FrontAxlePositionfromCG, b=VEH.RearAxlePositionfromCG, w=VEH.TrackWidth, figBorder=10, bufferSize=102400, pltDT=.1}
      mask prompts: a "Distance to front axle from CG, a [m]:"; b "Distance to rear axle from CG, b [m]:"; w "Track width, w [m]:"; figBorder "Distance to figure borders, figBorder [m]:"; bufferSize "Path buffer sampe size, bufferSize []:"; pltDT "Plot update rate, pltDT [s]:"
      mask help: This block will display a MATLAB figure which indicates the vehicle path, current position and heading velocity.
      mask TypeOptions a: Vehicle XY Plotter/a
      mask TypeOptions b: Vehicle XY Plotter/b
      mask TypeOptions w: Vehicle XY Plotter/w
      mask TypeOptions figBorder: Vehicle XY Plotter/figBorder
      mask TypeOptions bufferSize: Vehicle XY Plotter/bufferSize
  Yaw Rate and Steer : Scope  NumInputPorts=2
  wires:
  Bus Selector2/2 -> Terminator2/1  "<Brake>"
  Bus Selector/1 -> Unit Conversion4/1  "<EngSpd>"
  Cntrl/1 -> ISO 15037-1:2006/2(Cntrl), Bus Selector2/1
  Rate Transition2/1 -> Steer vs Ay/2
  Unit Conversion2/1 -> Signal Specification/1
  Bus Selector2/1 -> Terminator1/1  "<Accel>"
  Signal Specification/1 -> Yaw Rate and Steer/2, Rate Transition1/1, "Steer, Velocity, Lat Accel"/1  "SteerAngle"
  VehFdbk/1 -> Bus Selector3/1, Bus Selector/1, Vehicle XY Plotter/1(VehFdbk), 3D Engine/1(VehFdbk), ISO 15037-1:2006/1(VehFdbk)  "VehFdbk"
  Unit Conversion1/1 -> Signal Specification1/1
  Bus Selector/2 -> "Steer, Velocity, Lat Accel"/2, Unit Conversion1/1  "<xdot>"
  Bus Selector2/3 -> Unit Conversion2/1  "<Steer>"
  Signal Specification1/1 -> Terminator/1  "xdot_mph"
  Rate Transition1/1 -> Steer vs Ay/1
  Bus Selector/3 -> Rate Transition2/1, "Steer, Velocity, Lat Accel"/3  "<ay>"
  Unit Conversion4/1 -> Signal Specification3/1
  Signal Specification3/1 -> Terminator3/1  "Engine_rpm"
  Unit Conversion3/1 -> Signal Specification2/1
  Signal Specification2/1 -> Yaw Rate and Steer/1
  Bus Selector3/1 -> Unit Conversion3/1  "<r>"

== system Working_Dynamics_Sparkle/Environment/Ground Feedback ==
  note: 1) Add Subsystem or Model blocks as valid variant choices.
      | 2) You cannot connect blocks at this level. At simulation, connectivity is automatically
      | determined, based on the active variant and port name matching.
  Friction : Inport
  3D Engine : Subsystem  VariantControl=1
  Constant : Subsystem  VariantControl=0
  Ground : Outport

== system Working_Dynamics_Sparkle/Longitudinal Driver1/Subsystem ==
  VelRef : Inport
  VelFDBK : Inport  Port=2
  -4-0 : Saturate  Commented=on  UpperLimit=0  LowerLimit=-4  ZeroCross=off
  0-3 : Saturate  Commented=on  UpperLimit=3  LowerLimit=0  ZeroCross=off
  Blank Message1 : robotlib/Blank Message  messageClass=Message  entityType=std_msgs/Float64  messageType=std_msgs/Float64  SampleTime=inf
      settings: SourceProductBaseCode=RO
  Bus Assignment1 : BusAssignment  AssignedSignals=Data
  MATLAB Function : MATLAB Function  TreatAsAtomicUnit=on
  PID Controller : simulink/Continuous/PID Controller  Commented=on  Controller=PID  Form=Parallel  TimeDomain=Continuous-time  SampleTime=-1  IntegratorMethod=Forward Euler  FilterMethod=Forward Euler  ControllerParametersSource=internal  P=3  I=0.4  D=0.05  UseFilter=on  N=100  TunerSelectOption=Frequency Response Based  InitialConditionSource=internal  InitialConditionForIntegrator=0.0  InitialConditionForFilter=0.0  DifferentiatorICPrevScaledInput=0  ExternalReset=none  TrackingMode=off  Kt=1  LimitOutput=on  UpperSaturationLimit=inf  LowerSaturationLimit=0  LinearizeAsGain=off  AntiWindupMode=clamping  Kb=1  POutMin=[]  POutMax=[]  IOutMin=[]  IOutMax=[]  DOutMin=[]  DOutMax=[]  NOutMin=[]  NOutMax=[]  SumOutMin=[]  SumOutMax=[]  SaturationOutMin=[]  SaturationOutMax=[]  PParamMin=[]  PParamMax=[]  IParamMin=[]  IParamMax=[]  DParamMin=[]  DParamMax=[]  NParamMin=[]  NParamMax=[]  KbParamMin=[]  KbParamMax=[]  KtParamMin=[]  KtParamMax=[]  KbOutMin=[]  KbOutMax=[]  KtOutMin=[]  KtOutMax=[]  IntegratorOutMin=[]  IntegratorOutMax=[]  FilterOutMin=[]  FilterOutMax=[]  SumI1OutMin=[]  SumI1OutMax=[]  SumI2OutMin=[]  SumI2OutMax=[]  SumI3OutMin=[]  SumI3OutMax=[]  SumI4OutMin=[]  SumI4OutMax=[]  SumDOutMin=[]  SumDOutMax=[]  DifferentiatorOutMin=[]  DifferentiatorOutMax=[]  FilterDiffOutCoefMin=[]  FilterDiffOutCoefMax=[]  ReciprocalOutMin=[]  ReciprocalOutMax=[]  SumDenOutMin=[]  SumDenOutMax=[]  SumNumOutMin=[]  SumNumOutMax=[]  DivideOutMin=[]  DivideOutMax=[]  IntegratorContinuousStateAttributes=''  IntegratorStateMustResolveToSignalObject=off  IntegratorRTWStateStorageClass=Auto  FilterContinuousStateAttributes=''  FilterStateMustResolveToSignalObject=off  FilterRTWStateStorageClass=Auto  ParallelPVariant=InternalParameters  IdealPVariant=Disabled  IVariant=InternalParameters  DVariant=InternalParameters  IntegratorVariant=Continuous  SatVariant=Enabled  AWVariant=ContClampingParallel  PCopyVariant=Disabled  TRVariant=Disabled  FdbkBlocksVariant=Forward  IdealPFdbkVariant=Disabled  SatFdbkVariant=Disabled  DerivativeFilterVariant=ContFilter  NVariant=InternalParameters  NCopyVariant=Disabled  FilterICVariant=InternalICsFilter  IntegratorICVariant=InternalICs  ExternalResetVariant=Disabled  TRSumVariant=Passthrough  SumFdbkVariant=Disabled  SumVariant=Sum_PID
  Plus : Sum  Commented=on  Inputs=+-
  Publish1 : robotlib/Publish  topicSource=Specify your own  topic=/catvehicle/v_error  messageType=std_msgs/Float64  messageQueueLength=1
      settings: SourceProductBaseCode=RO
  Unary Minus : UnaryMinus  Commented=on
  Accel : Outport  Unit=m/s^2
  Decel : Outport  Port=2  Unit=m/s^2
  wires:
  MATLAB Function/3(accel_in) -> Accel/1  "Accel"
  -4-0/1 -> Unary Minus/1
  VelFDBK/1 -> MATLAB Function/2(vel_feedback)
  VelRef/1 -> MATLAB Function/1(vel_ref)
  PID Controller/1 -> 0-3/1, -4-0/1  "Cmd"
  Plus/1 -> PID Controller/1
  Bus Assignment1/1 -> Publish1/1
  Blank Message1/1 -> Bus Assignment1/1
  MATLAB Function/2(brake_in) -> Decel/1
  MATLAB Function/1(v_error) -> Bus Assignment1/2

== system Working_Dynamics_Sparkle/Passenger Vehicle/Subsystem ==
  Env : Inport
  Driveline : Inport  Port=2
  Bus Selector1 : BusSelector  OutputSignals=Gnd.z.G_FL_z,Gnd.z.G_FR_z,Gnd.z.G_RL_z,Gnd.z.G_RR_z
  Bus Selector2 : BusSelector  OutputSignals=Wind
  Bus Selector3 : BusSelector  OutputSignals=Gnd.mu.mu_FL,Gnd.mu.mu_FR,Gnd.mu.mu_RL,Gnd.mu.mu_RR
  Bus Selector4 : BusSelector  OutputSignals=WhlAng,AxlTrq,BrkPrs
  Vector Concatenate : Concatenate  NumInputs=4
  Vector Concatenate1 : Concatenate  NumInputs=4
  Wind : Outport
  Gnd : Outport  Port=2
  mu : Outport  Port=3
  WhlAng : Outport  Port=4
  AxleTrq : Outport  Port=5
  BrkPrs : Outport  Port=6
  wires:
  Env/1 -> Bus Selector3/1, Bus Selector1/1, Bus Selector2/1
  Bus Selector2/1 -> Wind/1  "<Wind>"
  Bus Selector3/1 -> Vector Concatenate/1  "<mu_FL>"
  Bus Selector3/2 -> Vector Concatenate/2  "<mu_FR>"
  Bus Selector3/3 -> Vector Concatenate/3  "<mu_RL>"
  Bus Selector3/4 -> Vector Concatenate/4  "<mu_RR>"
  Vector Concatenate/1 -> mu/1
  Bus Selector1/1 -> Vector Concatenate1/1  "<G_FL_z>"
  Bus Selector1/2 -> Vector Concatenate1/2  "<G_FR_z>"
  Bus Selector1/3 -> Vector Concatenate1/3  "<G_RL_z>"
  Bus Selector1/4 -> Vector Concatenate1/4  "<G_RR_z>"
  Vector Concatenate1/1 -> Gnd/1
  Driveline/1 -> Bus Selector4/1
  Bus Selector4/2 -> AxleTrq/1  "<AxlTrq>"
  Bus Selector4/1 -> WhlAng/1  "<WhlAng>"
  Bus Selector4/3 -> BrkPrs/1  "<BrkPrs>"

== system Working_Dynamics_Sparkle/Passenger Vehicle/Subsystem1 ==
  WhlAng : Inport
  AxlTrq : Inport  Port=2
  BrkPrs : Inport  Port=3
  EngSpd : Inport  Port=4
  PropShftSpd : Inport  Port=5
  StrWhlTrq : Inport  Port=6
  Bus Creator1 : BusCreator  Inputs=5
  Bus Creator2 : BusCreator  Inputs=1
  Driveline : Outport
  Steering : Outport  Port=2
  wires:
  Bus Creator1/1 -> Driveline/1  "Driveline"
  PropShftSpd/1 -> Bus Creator1/5  "PropShftSpd"
  AxlTrq/1 -> Bus Creator1/2  "AxlTrq"
  WhlAng/1 -> Bus Creator1/1  "WhlAng"
  EngSpd/1 -> Bus Creator1/4  "EngSpd"
  BrkPrs/1 -> Bus Creator1/3  "BrkPrs"
  StrWhlTrq/1 -> Bus Creator2/1  "StrWhlTrq"
  Bus Creator2/1 -> Steering/1  "Steering"

== system Working_Dynamics_Sparkle/Passenger Vehicle/Subsystem2 ==
  Cntrl : Inport
  SteerCmd : Inport  Port=2
  EngTrqCmd : Inport  Port=3
  Wheels : Inport  Port=4
  Bus Selector1 : BusSelector  OutputSignals=Steer
  Bus Selector2 : BusSelector  OutputSignals=omega
  Bus Selector3 : BusSelector  OutputSignals=Transmission.GearCmd,Brake.PrsCmd,Diff.PrsCmd
  Bus Selector4 : BusSelector  OutputSignals=EngTrq
  Steer : Outport
  EngTrq : Outport  Port=2
  GearCmd : Outport  Port=3
  PrsCmd : Outport  Port=4
  omega : Outport  Port=5
  DiffPrsCmd : Outport  Port=6
  wires:
  Cntrl/1 -> Bus Selector3/1
  Bus Selector3/1 -> GearCmd/1  "<GearCmd>"
  SteerCmd/1 -> Bus Selector1/1
  Wheels/1 -> Bus Selector2/1
  Bus Selector2/1 -> omega/1  "<omega>"
  Bus Selector3/2 -> PrsCmd/1  "<PrsCmd>"
  EngTrqCmd/1 -> Bus Selector4/1
  Bus Selector1/1 -> Steer/1  "<Steer>"
  Bus Selector4/1 -> EngTrq/1  "<EngTrq>"
  Bus Selector3/3 -> DiffPrsCmd/1  "<PrsCmd>"

== system Working_Dynamics_Sparkle/Passenger Vehicle/Subsystem3 ==
  Cntrl : Inport
  Driveline : Inport  Port=2
  Bus Selector : BusSelector  OutputSignals=ECU.EngTrqCmd
  Bus Selector1 : BusSelector  OutputSignals=EngSpd
  EngTrqCmd : Outport
  EngSpd : Outport  Port=2
  wires:
  Driveline/1 -> Bus Selector1/1
  Cntrl/1 -> Bus Selector/1
  Bus Selector/1 -> EngTrqCmd/1  "<EngTrqCmd>"
  Bus Selector1/1 -> EngSpd/1  "<EngSpd>"

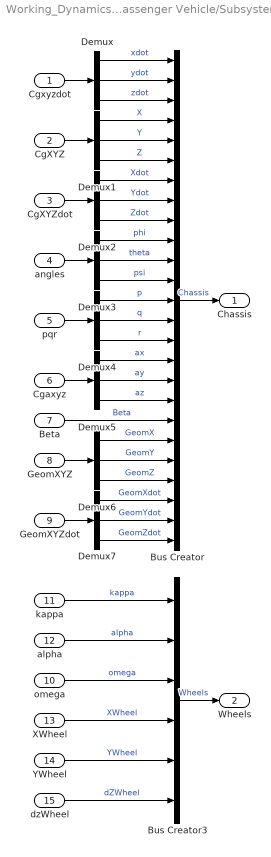
== system Working_Dynamics_Sparkle/Passenger Vehicle/Subsystem4 ==
  Cgxyzdot : Inport
  CgXYZ : Inport  Port=2
  CgXYZdot : Inport  Port=3
  angles : Inport  Port=4
  pqr : Inport  Port=5
  Cgaxyz : Inport  Port=6
  Beta : Inport  Port=7
  GeomXYZ : Inport  Port=8
  GeomXYZdot : Inport  Port=9
  omega : Inport  Port=10
  kappa : Inport  Port=11
  alpha : Inport  Port=12
  XWheel : Inport  Port=13
  YWheel : Inport  Port=14
  dzWheel : Inport  Port=15
  Bus Creator : BusCreator  Inputs=25
  Bus Creator3 : BusCreator  Inputs=6
  Demux{,1..7} (8 alike) : Demux  Outputs=3
  Chassis : Outport
  Wheels : Outport  Port=2
  wires:
  Bus Creator/1 -> Chassis/1  "Chassis"
  omega/1 -> Bus Creator3/3  "omega"
  dzWheel/1 -> Bus Creator3/6  "dZWheel"
  kappa/1 -> Bus Creator3/1  "kappa"
  Bus Creator3/1 -> Wheels/1  "Wheels"
  YWheel/1 -> Bus Creator3/5  "YWheel"
  XWheel/1 -> Bus Creator3/4  "XWheel"
  alpha/1 -> Bus Creator3/2  "alpha"
  Cgxyzdot/1 -> Demux/1
  CgXYZ/1 -> Demux1/1
  CgXYZdot/1 -> Demux2/1
  angles/1 -> Demux3/1
  pqr/1 -> Demux4/1
  Cgaxyz/1 -> Demux5/1
  GeomXYZdot/1 -> Demux7/1
  GeomXYZ/1 -> Demux6/1
  Demux/1 -> Bus Creator/1  "xdot"
  Demux/2 -> Bus Creator/2  "ydot"
  Demux/3 -> Bus Creator/3  "zdot"
  Demux1/1 -> Bus Creator/4  "X"
  Demux1/2 -> Bus Creator/5  "Y"
  Demux1/3 -> Bus Creator/6  "Z"
  Demux2/1 -> Bus Creator/7  "Xdot"
  Demux2/2 -> Bus Creator/8  "Ydot"
  Demux2/3 -> Bus Creator/9  "Zdot"
  Demux3/1 -> Bus Creator/10  "phi"
  Demux3/2 -> Bus Creator/11  "theta"
  Demux3/3 -> Bus Creator/12  "psi"
  Demux4/1 -> Bus Creator/13  "p"
  Demux4/2 -> Bus Creator/14  "q"
  Demux4/3 -> Bus Creator/15  "r"
  Demux5/1 -> Bus Creator/16  "ax"
  Demux5/2 -> Bus Creator/17  "ay"
  Demux5/3 -> Bus Creator/18  "az"
  Beta/1 -> Bus Creator/19  "Beta"
  Demux6/1 -> Bus Creator/20  "GeomX"
  Demux6/2 -> Bus Creator/21  "GeomY"
  Demux6/3 -> Bus Creator/22  "GeomZ"
  Demux7/1 -> Bus Creator/23  "GeomXdot"
  Demux7/2 -> Bus Creator/24  "GeomYdot"
  Demux7/3 -> Bus Creator/25  "GeomZdot"

== system Working_Dynamics_Sparkle/Passenger Vehicle/Subsystem5 ==
  "EngTrq " : Inport
  Bus Creator : BusCreator  Inputs=1
  Eng : Outport
  wires:
  "EngTrq "/1 -> Bus Creator/1  "EngTrq"
  Bus Creator/1 -> Eng/1

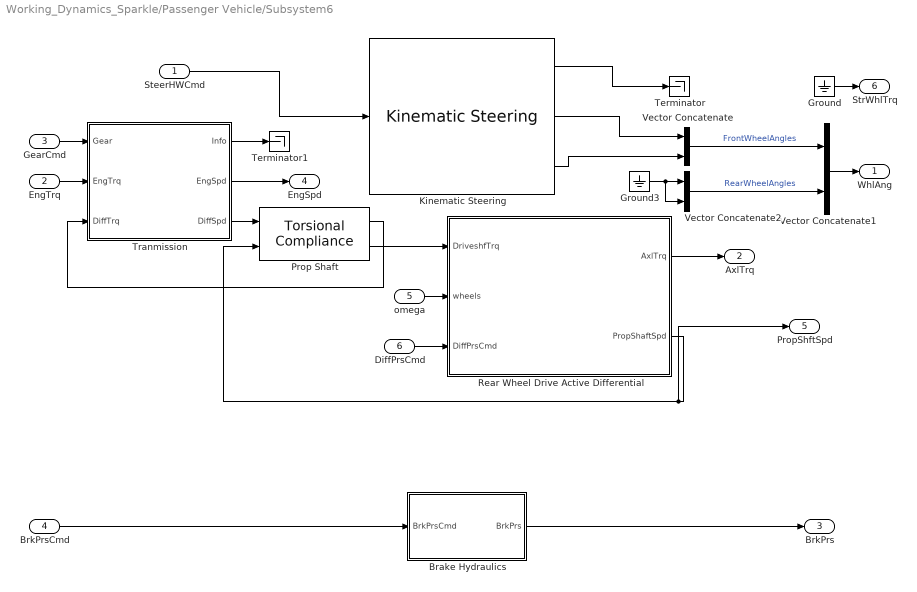
== system Working_Dynamics_Sparkle/Passenger Vehicle/Subsystem6 ==
  SteerHWCmd : Inport
  EngTrq : Inport  Port=2
  GearCmd : Inport  Port=3
  BrkPrsCmd : Inport  Port=4  PortDimensions=4
  omega : Inport  Port=5
  DiffPrsCmd : Inport  Port=6
  Brake Hydraulics : Subsystem
  Ground : Ground
  Ground3 : Ground
  Kinematic Steering : vehdynlibsteering/Kinematic Steering  StrgType=Ackerman  StrgRatioType=Constant  Loc=Front  NrmlFctr=1  TrckWdth=1.922  WhlBase=(1.515+1.504)  Db=0  StrgRng=3*pi  StrgAngBpts="[-6.2832   -5.0265   -3.7699   -2.5133   -1.2566         0    1.2566    2.5133    3.7699    5.0265    6.2832]"  StrgRatioTbl=|  StrgRatio=18  StrgArmLngth=0.1  RckCsLngth=0.5  TieRodLngth=0.248  D=0.2  PnnRadius=0.0057  PnnRadiusTbl="[0.0055    0.0055    0.0056    0.0057    0.0058    0.0057    0.0057    0.0057    0.0056    0.0055    0.0055]"  RodLngth=0.1  ParaArmLngth=0.9  aMode=2
      | [13.5000   13.3750   13.2500   13.1250   13.0000   13.0000   13.0000   13.1250   13.2500   13.3750   13.5000
      | ]
      settings: SourceProductName=Vehicle Dynamics Blockset
  Prop Shaft : autolibsharedcoupling/Torsional Compliance  port_config=Simulink  k=5e3  b=100  theta_o=0  domega_o=0  omega_c=150  blkID=0  aMode=2
      settings: SourceProductName=Powertrain Blockset  SourceProductBaseCode=PW
  Rear Wheel Drive Active Differential : Subsystem
  Terminator : Terminator
  Terminator1 : Terminator
  Tranmission : Subsystem
  Vector Concatenate : Concatenate
  Vector Concatenate1 : Concatenate
  Vector Concatenate2 : Concatenate
  WhlAng : Outport  Unit=rad
  AxlTrq : Outport  Port=2
  BrkPrs : Outport  Port=3  PortDimensions=4
  EngSpd : Outport  Port=4
  PropShftSpd : Outport  Port=5
  StrWhlTrq : Outport  Port=6  Unit=N*m
  wires:
  Vector Concatenate1/1 -> WhlAng/1
  Vector Concatenate/1 -> Vector Concatenate1/1  "FrontWheelAngles"
  Tranmission/2(EngSpd) -> EngSpd/1
  Rear Wheel Drive Active Differential/1(AxlTrq) -> AxlTrq/1
  omega/1 -> Rear Wheel Drive Active Differential/2(wheels)
  Kinematic Steering/2 -> Vector Concatenate/1
  Ground3/1 -> Vector Concatenate2/2, Vector Concatenate2/1
  Prop Shaft/1 -> Tranmission/3(DiffTrq)
  Kinematic Steering/3 -> Vector Concatenate/2
  Rear Wheel Drive Active Differential/2(PropShaftSpd) -> PropShftSpd/1, Prop Shaft/2
  SteerHWCmd/1 -> Kinematic Steering/1
  DiffPrsCmd/1 -> Rear Wheel Drive Active Differential/3(DiffPrsCmd)
  Tranmission/3(DiffSpd) -> Prop Shaft/1
  Ground/1 -> StrWhlTrq/1
  Tranmission/1(Info) -> Terminator1/1
  Prop Shaft/2 -> Rear Wheel Drive Active Differential/1(DriveshfTrq)
  Brake Hydraulics/1(BrkPrs) -> BrkPrs/1
  GearCmd/1 -> Tranmission/1(Gear)
  BrkPrsCmd/1 -> Brake Hydraulics/1(BrkPrsCmd)
  Vector Concatenate2/1 -> Vector Concatenate1/2  "RearWheelAngles"
  Kinematic Steering/1 -> Terminator/1
  EngTrq/1 -> Tranmission/2(EngTrq)

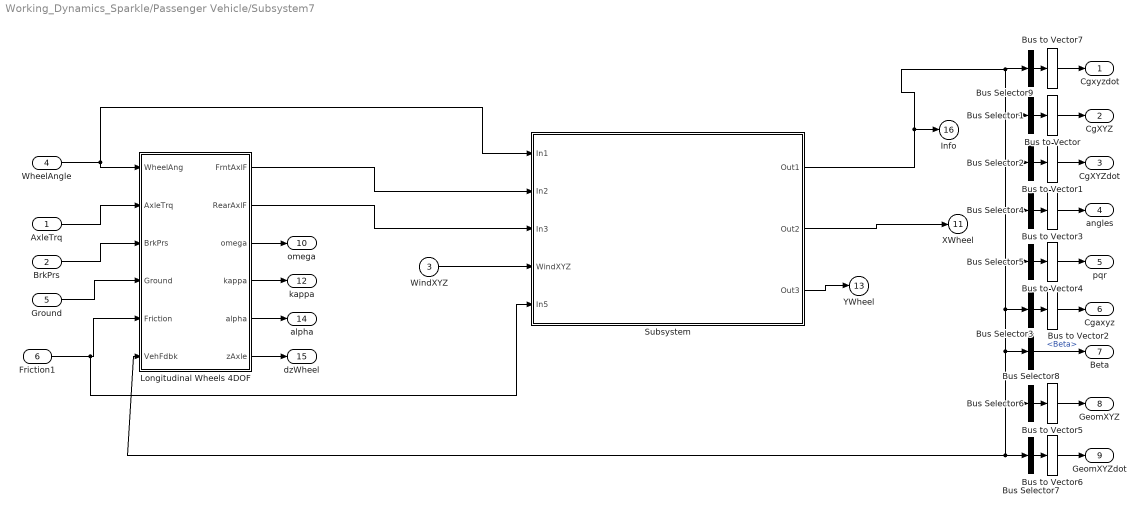
== system Working_Dynamics_Sparkle/Passenger Vehicle/Subsystem7 ==
  AxleTrq : Inport  Unit=N*m  PortDimensions=4
  BrkPrs : Inport  Port=2  Unit=Pa  PortDimensions=4
  WindXYZ : Inport  Port=3
  WheelAngle : Inport  Port=4  Unit=rad  PortDimensions=4
  Ground : Inport  Port=5  Unit=m  PortDimensions=4
  Friction1 : Inport  Port=6  Unit=1  PortDimensions=4
  Bus Selector1 : BusSelector  OutputSignals=InertFrm.Cg.Disp.X,InertFrm.Cg.Disp.Y,InertFrm.Cg.Disp.Z  OutputAsBus=on
  Bus Selector2 : BusSelector  OutputSignals=InertFrm.Cg.Vel.Xdot,InertFrm.Cg.Vel.Ydot,InertFrm.Cg.Vel.Zdot  OutputAsBus=on
  Bus Selector3 : BusSelector  OutputSignals=BdyFrm.Cg.Acc.ax,BdyFrm.Cg.Acc.ay,BdyFrm.Cg.Acc.az  OutputAsBus=on
  Bus Selector4 : BusSelector  OutputSignals=InertFrm.Cg.Ang.phi,InertFrm.Cg.Ang.theta,InertFrm.Cg.Ang.psi  OutputAsBus=on
  Bus Selector5 : BusSelector  OutputSignals=BdyFrm.Cg.AngVel.p,BdyFrm.Cg.AngVel.q,BdyFrm.Cg.AngVel.r  OutputAsBus=on
  Bus Selector6 : BusSelector  OutputSignals=InertFrm.Geom.Disp.X,InertFrm.Geom.Disp.Y,InertFrm.Geom.Disp.Z  OutputAsBus=on
  Bus Selector7 : BusSelector  OutputSignals=InertFrm.Geom.Vel.Xdot,InertFrm.Geom.Vel.Ydot,InertFrm.Geom.Vel.Zdot  OutputAsBus=on
  Bus Selector8 : BusSelector  OutputSignals=BdyFrm.Geom.Ang.Beta
  Bus Selector9 : BusSelector  OutputSignals=BdyFrm.Cg.Vel.xdot,BdyFrm.Cg.Vel.ydot,BdyFrm.Cg.Vel.zdot  OutputAsBus=on
  Bus to Vector{,1..7} (8 alike) : BusToVector
  Longitudinal Wheels 4DOF : Subsystem  VariantControl=1  mask{wheelMode=Single track (bicycle)}
      mask prompts: wheelMode "Wheel mode:"
      settings: AttributesFormatString=%<wheelMode>
      mask TypeOptions wheelMode: Single track (bicycle) | Dual track
      mask Callback wheelMode:
      | switch get_param(gcb,'wheelMode')
      |     case 'Single track (bicycle)'
      |         set_param([bdroot '/Longitudinal Wheels 4DOF/Velocity and Vertical Load'],'OverrideUsingVariant','0')
      |         set_param([bdroot '/Longitudinal Wheels 4DOF/Axle Forces'],'OverrideUsingVariant','0')
      |     case 'Dual track'
      |         set_param([bdroot '/Longitudinal Wheels 4DOF/Velocity and Vertical Load'],'OverrideUsingVariant','1')
      |         set_param([bdroot '/Longitudinal Wheels 4DOF/Axle Forces'],'OverrideUsingVariant','1')
      |     otherwise
      |         set_param([bdroot '/Longitudinal Wheels 4DOF/Velocity and Vertical Load'],'OverrideUsingVariant','0')
      |         set_param([bdroot '/Longitudinal Wheels 4DOF/Axle Forces'],'OverrideUsingVariant','0')
      | end
  Subsystem : Subsystem
  Cgxyzdot : Outport
  CgXYZ : Outport  Port=2
  CgXYZdot : Outport  Port=3
  angles : Outport  Port=4
  pqr : Outport  Port=5
  Cgaxyz : Outport  Port=6
  Beta : Outport  Port=7
  GeomXYZ : Outport  Port=8
  GeomXYZdot : Outport  Port=9  Unit=m/s
  omega : Outport  Port=10  PortDimensions=4
  XWheel : Outport  Port=11  Unit=m
  kappa : Outport  Port=12  PortDimensions=4
  " YWheel" : Outport  Port=13  Unit=m
  alpha : Outport  Port=14  PortDimensions=4
  dzWheel : Outport  Port=15
  " Info" : Outport  Port=16
  wires:
  Bus to Vector1/1 -> CgXYZdot/1
  Ground/1 -> Longitudinal Wheels 4DOF/4(Ground)
  Longitudinal Wheels 4DOF/6(zAxle) -> dzWheel/1
  Bus to Vector4/1 -> pqr/1
  Longitudinal Wheels 4DOF/3(omega) -> omega/1
  Bus to Vector6/1 -> GeomXYZdot/1
  Bus Selector2/1 -> Bus to Vector1/1
  Longitudinal Wheels 4DOF/5(alpha) -> alpha/1
  Bus Selector1/1 -> Bus to Vector/1
  Bus to Vector5/1 -> GeomXYZ/1
  Bus Selector4/1 -> Bus to Vector3/1
  Bus Selector3/1 -> Bus to Vector2/1
  Bus to Vector3/1 -> angles/1
  Bus to Vector7/1 -> Cgxyzdot/1
  Bus Selector9/1 -> Bus to Vector7/1
  AxleTrq/1 -> Longitudinal Wheels 4DOF/2(AxleTrq)
  BrkPrs/1 -> Longitudinal Wheels 4DOF/3(BrkPrs)
  WheelAngle/1 -> Subsystem/1(In1), Longitudinal Wheels 4DOF/1(WheelAng)
  Bus Selector6/1 -> Bus to Vector5/1
  Longitudinal Wheels 4DOF/4(kappa) -> kappa/1
  Bus to Vector2/1 -> Cgaxyz/1
  Bus to Vector/1 -> CgXYZ/1
  Bus Selector7/1 -> Bus to Vector6/1
  Bus Selector5/1 -> Bus to Vector4/1
  Friction1/1 -> Subsystem/5(In5), Longitudinal Wheels 4DOF/5(Friction)
  Bus Selector8/1 -> Beta/1  "<Beta>"
  Subsystem/1(Out1) -> Bus Selector8/1, Bus Selector6/1, Longitudinal Wheels 4DOF/6(VehFdbk), Bus Selector7/1, Bus Selector3/1, Bus Selector5/1, Bus Selector4/1, Bus Selector2/1, Bus Selector1/1, Bus Selector9/1, " Info"/1
  Longitudinal Wheels 4DOF/1(FrntAxlF) -> Subsystem/2(In2)
  Longitudinal Wheels 4DOF/2(RearAxlF) -> Subsystem/3(In3)
  WindXYZ/1 -> Subsystem/4(WindXYZ)
  Subsystem/2(Out2) -> XWheel/1
  Subsystem/3(Out3) -> " YWheel"/1
